simulink model "PC_Quadcopter_Simulation"  (R2020b)
settings: Solver=ode45  StartTime=0.0  StopTime=10  FixedStep=0.05  MaxStep=0.06  RelTol=1e-3  EnableMultiTasking=on
model workspace (MAT data in the model file):
  Sig : Simulink.Signal (value not decoded)
undefined symbols (not defined in the file): IC, quadModel
libraries: pid_lib x9, simulink x6, shared6dof x1
(part 2 of 2)

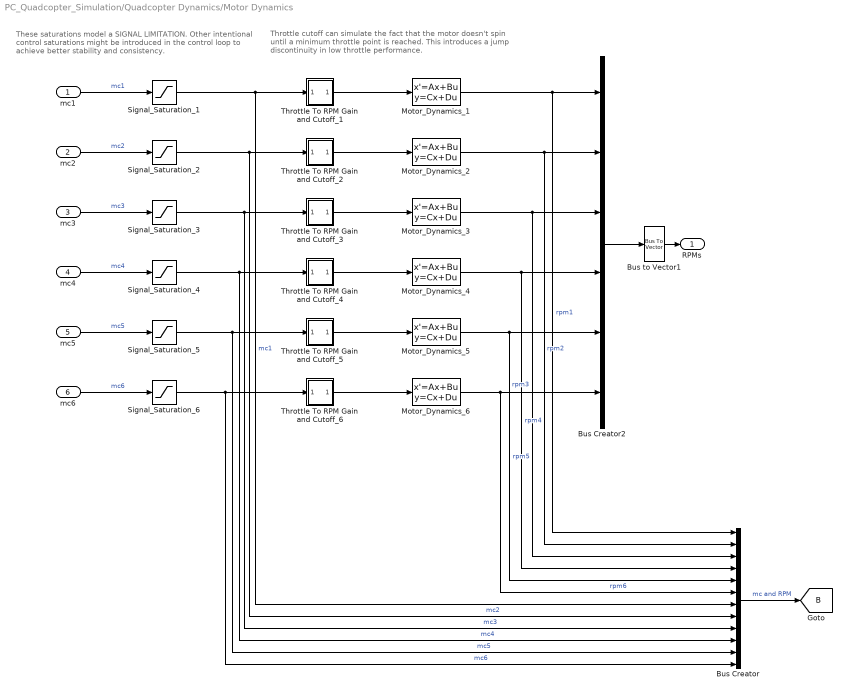
== system PC_Quadcopter_Simulation/Quadcopter Dynamics/Motor Dynamics ==
  note: Throttle cutoff can simulate the fact that the motor doesn't
      | spin until a minimum throttle point is reached. This introduces
      | a jump discontinuity in low throttle performance.
  note: These saturations model a SIGNAL LIMITATION.
      | Other intentional control saturations might be introduced in the
      | control loop to achieve better stability and consistency.
  mc1 : Inport
  mc2 : Inport  Port=2
  mc3 : Inport  Port=3
  mc4 : Inport  Port=4
  mc5 : Inport  Port=5
  mc6 : Inport  Port=6
  Bus Creator : BusCreator  Inputs=12
  Bus Creator2 : BusCreator  Inputs=6
  Bus to Vector1 : BusToVector
  Motor_Dynamics_1 : StateSpace  A=-1/quadModel.T  C=1/quadModel.T  D=0  InitialCondition=IC.w1*quadModel.T
  Motor_Dynamics_2 : StateSpace  A=-1/quadModel.T  C=1/quadModel.T  D=0  InitialCondition=IC.w2*quadModel.T
  Motor_Dynamics_3 : StateSpace  A=-1/quadModel.T  C=1/quadModel.T  D=0  InitialCondition=IC.w3*quadModel.T
  Motor_Dynamics_4 : StateSpace  A=-1/quadModel.T  C=1/quadModel.T  D=0  InitialCondition=IC.w4*quadModel.T
  Motor_Dynamics_5 : StateSpace  A=-1/quadModel.T  C=1/quadModel.T  D=0  InitialCondition=IC.w4*quadModel.T
  Motor_Dynamics_6 : StateSpace  A=-1/quadModel.T  C=1/quadModel.T  D=0  InitialCondition=IC.w4*quadModel.T
  Signal_Saturation_{1..6} (6 alike) : Saturate  UpperLimit=100  LowerLimit=0
  Throttle To RPM Gain and Cutoff_1 : Subsystem
  Throttle To RPM Gain and Cutoff_2 : Subsystem
  Throttle To RPM Gain and Cutoff_3 : Subsystem
  Throttle To RPM Gain and Cutoff_4 : Subsystem
  Throttle To RPM Gain and Cutoff_5 : Subsystem
  Throttle To RPM Gain and Cutoff_6 : Subsystem
  RPMs : Outport
  tag scope: B=global
  wires:
  mc1/1 -> Signal_Saturation_1/1  "mc1"
  mc2/1 -> Signal_Saturation_2/1  "mc2"
  mc3/1 -> Signal_Saturation_3/1  "mc3"
  mc4/1 -> Signal_Saturation_4/1  "mc4"
  Throttle To RPM Gain and Cutoff_1/1(Out5) -> Motor_Dynamics_1/1
  Throttle To RPM Gain and Cutoff_2/1(Out5) -> Motor_Dynamics_2/1
  Throttle To RPM Gain and Cutoff_3/1(Out5) -> Motor_Dynamics_3/1
  Throttle To RPM Gain and Cutoff_4/1(Out5) -> Motor_Dynamics_4/1
  Motor_Dynamics_1/1 -> Bus Creator/1, Bus Creator2/1  "rpm1"
  Motor_Dynamics_2/1 -> Bus Creator/2, Bus Creator2/2  "rpm2"
  Motor_Dynamics_3/1 -> Bus Creator/3, Bus Creator2/3  "rpm3"
  Motor_Dynamics_4/1 -> Bus Creator/4, Bus Creator2/4  "rpm4"
  Bus Creator/1 -> [B]  "mc and RPM"
  mc5/1 -> Signal_Saturation_5/1  "mc5"
  Throttle To RPM Gain and Cutoff_5/1(Out5) -> Motor_Dynamics_5/1
  mc6/1 -> Signal_Saturation_6/1  "mc6"
  Throttle To RPM Gain and Cutoff_6/1(Out5) -> Motor_Dynamics_6/1
  Motor_Dynamics_6/1 -> Bus Creator/6, Bus Creator2/6  "rpm6"
  Motor_Dynamics_5/1 -> Bus Creator/5, Bus Creator2/5  "rpm5"
  Signal_Saturation_3/1 -> Bus Creator/9, Throttle To RPM Gain and Cutoff_3/1(In5)  "mc3"
  Signal_Saturation_4/1 -> Bus Creator/10, Throttle To RPM Gain and Cutoff_4/1(In5)  "mc4"
  Signal_Saturation_1/1 -> Bus Creator/7, Throttle To RPM Gain and Cutoff_1/1(In5)  "mc1"
  Signal_Saturation_5/1 -> Bus Creator/11, Throttle To RPM Gain and Cutoff_5/1(In5)  "mc5"
  Signal_Saturation_6/1 -> Bus Creator/12, Throttle To RPM Gain and Cutoff_6/1(In5)  "mc6"
  Signal_Saturation_2/1 -> Bus Creator/8, Throttle To RPM Gain and Cutoff_2/1(In5)  "mc2"
  Bus Creator2/1 -> Bus to Vector1/1
  Bus to Vector1/1 -> RPMs/1

== system PC_Quadcopter_Simulation/Quadcopter Dynamics/Subsystem ==
  RPMs : Inport
  States : Inport  Port=2
  DCM : Inport  Port=3
  Forces : Subsystem
  Moments : Subsystem
  ForceOut : Outport
  MomentOut : Outport  Port=2
  wires:
  RPMs/1 -> Moments/2(RPMs), Forces/1(RPMs)  "RPMs"
  Forces/1(Forces) -> ForceOut/1
  States/1 -> Moments/1(States)  "States"
  Moments/1(Moments) -> MomentOut/1
  DCM/1 -> Forces/2(DCM)

== system PC_Quadcopter_Simulation/Quadcopter Dynamics/Motor Dynamics/Throttle To RPM Gain and Cutoff_1 ==
  note: minThr should be a quad.mat value
  note: This gain should be a quad.mat value
  note: This constant should be a quad.mat value
  note: Output equals linearly scaled RPM
      | for given throttle input if throttle input >=Throttle Cuttoff (minThr)
      | else output is zero.
  In5 : Inport
  Constant : Constant  Value=quadModel.b
  Gain : Gain  Gain=quadModel.cr
  Minimum Throttle Cutoff : simulink/Logic and Bit Operations/Compare To Constant  relop=>=  const=quadModel.minThr  OutDataTypeStr=uint8
  Product : Product
  Sum1 : Sum  Inputs=++|
  Out5 : Outport
  wires:
  Minimum Throttle Cutoff/1 -> Product/2
  Product/1 -> Out5/1
  In5/1 -> Gain/1, Minimum Throttle Cutoff/1
  Gain/1 -> Sum1/2
  Sum1/1 -> Product/1
  Constant/1 -> Sum1/1

== system PC_Quadcopter_Simulation/Quadcopter Dynamics/Motor Dynamics/Throttle To RPM Gain and Cutoff_2 ==
  note: minThr should be a quad.mat value
  note: This gain should be a quad.mat value
  note: This constant should be a quad.mat value
  note: Output equals linearly scaled RPM
      | for given throttle input if throttle input >=Throttle Cuttoff (minThr)
      | else output is zero.
  In5 : Inport
  Constant : Constant  Value=quadModel.b
  Gain : Gain  Gain=quadModel.cr
  Minimum Throttle Cutoff : simulink/Logic and Bit Operations/Compare To Constant  relop=>=  const=quadModel.minThr  OutDataTypeStr=uint8
  Product : Product
  Sum1 : Sum  Inputs=++|
  Out5 : Outport
  wires:
  Minimum Throttle Cutoff/1 -> Product/2
  Product/1 -> Out5/1
  In5/1 -> Gain/1, Minimum Throttle Cutoff/1
  Gain/1 -> Sum1/2
  Sum1/1 -> Product/1
  Constant/1 -> Sum1/1

== system PC_Quadcopter_Simulation/Quadcopter Dynamics/Motor Dynamics/Throttle To RPM Gain and Cutoff_3 ==
  note: minThr should be a quad.mat value
  note: This gain should be a quad.mat value
  note: This constant should be a quad.mat value
  note: Output equals linearly scaled RPM
      | for given throttle input if throttle input >=Throttle Cuttoff (minThr)
      | else output is zero.
  In5 : Inport
  Constant : Constant  Value=quadModel.b
  Gain : Gain  Gain=quadModel.cr
  Minimum Throttle Cutoff : simulink/Logic and Bit Operations/Compare To Constant  relop=>=  const=quadModel.minThr  OutDataTypeStr=uint8
  Product : Product
  Sum1 : Sum  Inputs=++|
  Out5 : Outport
  wires:
  Minimum Throttle Cutoff/1 -> Product/2
  Product/1 -> Out5/1
  In5/1 -> Gain/1, Minimum Throttle Cutoff/1
  Gain/1 -> Sum1/2
  Sum1/1 -> Product/1
  Constant/1 -> Sum1/1

== system PC_Quadcopter_Simulation/Quadcopter Dynamics/Motor Dynamics/Throttle To RPM Gain and Cutoff_4 ==
  note: minThr should be a quad.mat value
  note: This gain should be a quad.mat value
  note: This constant should be a quad.mat value
  note: Output equals linearly scaled RPM
      | for given throttle input if throttle input >=Throttle Cuttoff (minThr)
      | else output is zero.
  In5 : Inport
  Constant : Constant  Value=quadModel.b
  Gain : Gain  Gain=quadModel.cr
  Minimum Throttle Cutoff : simulink/Logic and Bit Operations/Compare To Constant  relop=>=  const=quadModel.minThr  OutDataTypeStr=uint8
  Product : Product
  Sum1 : Sum  Inputs=++|
  Out5 : Outport
  wires:
  Minimum Throttle Cutoff/1 -> Product/2
  Product/1 -> Out5/1
  In5/1 -> Gain/1, Minimum Throttle Cutoff/1
  Gain/1 -> Sum1/2
  Sum1/1 -> Product/1
  Constant/1 -> Sum1/1

== system PC_Quadcopter_Simulation/Quadcopter Dynamics/Motor Dynamics/Throttle To RPM Gain and Cutoff_5 ==
  note: minThr should be a quad.mat value
  note: This gain should be a quad.mat value
  note: This constant should be a quad.mat value
  note: Output equals linearly scaled RPM
      | for given throttle input if throttle input >=Throttle Cuttoff (minThr)
      | else output is zero.
  In5 : Inport
  Constant : Constant  Value=quadModel.b
  Gain : Gain  Gain=quadModel.cr
  Minimum Throttle Cutoff : simulink/Logic and Bit Operations/Compare To Constant  relop=>=  const=quadModel.minThr  OutDataTypeStr=uint8
  Product : Product
  Sum1 : Sum  Inputs=++|
  Out5 : Outport
  wires:
  Minimum Throttle Cutoff/1 -> Product/2
  Product/1 -> Out5/1
  In5/1 -> Gain/1, Minimum Throttle Cutoff/1
  Gain/1 -> Sum1/2
  Sum1/1 -> Product/1
  Constant/1 -> Sum1/1

== system PC_Quadcopter_Simulation/Quadcopter Dynamics/Motor Dynamics/Throttle To RPM Gain and Cutoff_6 ==
  note: minThr should be a quad.mat value
  note: This gain should be a quad.mat value
  note: This constant should be a quad.mat value
  note: Output equals linearly scaled RPM
      | for given throttle input if throttle input >=Throttle Cuttoff (minThr)
      | else output is zero.
  In5 : Inport
  Constant : Constant  Value=quadModel.b
  Gain : Gain  Gain=quadModel.cr
  Minimum Throttle Cutoff : simulink/Logic and Bit Operations/Compare To Constant  relop=>=  const=quadModel.minThr  OutDataTypeStr=uint8
  Product : Product
  Sum1 : Sum  Inputs=++|
  Out5 : Outport
  wires:
  Minimum Throttle Cutoff/1 -> Product/2
  Product/1 -> Out5/1
  In5/1 -> Gain/1, Minimum Throttle Cutoff/1
  Gain/1 -> Sum1/2
  Sum1/1 -> Product/1
  Constant/1 -> Sum1/1

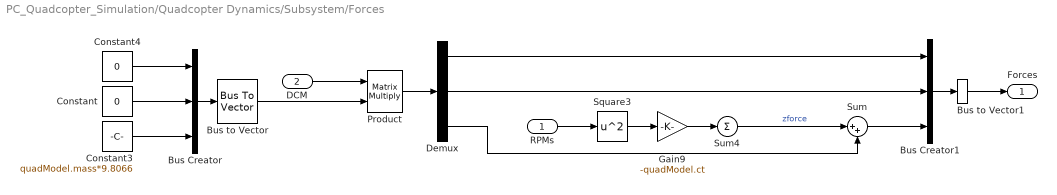
== system PC_Quadcopter_Simulation/Quadcopter Dynamics/Subsystem/Forces ==
  RPMs : Inport
  DCM : Inport  Port=2
  Bus Creator : BusCreator  Inputs=3
  Bus Creator1 : BusCreator  Inputs=3
  Bus to Vector : BusToVector
  Bus to Vector1 : BusToVector
  Constant : Constant  Value=0
  Constant3 : Constant  Value=quadModel.mass*9.8066
  Constant4 : Constant  Value=0
  Demux : Demux  Outputs=3
  Gain9 : Gain  Gain=-quadModel.ct
  Product : Product  Multiplication=Matrix(*)
  Square3 : Math  Operator=square  SaturateOnIntegerOverflow=on
  Sum : Sum  Inputs=|++
  Sum4 : Sum  Inputs=+
  Forces : Outport
  wires:
  Demux/2 -> Bus Creator1/2
  Bus Creator1/1 -> Bus to Vector1/1
  Demux/1 -> Bus Creator1/1
  Gain9/1 -> Sum4/1
  Bus to Vector1/1 -> Forces/1
  Square3/1 -> Gain9/1
  Sum4/1 -> Sum/1  "zforce"
  RPMs/1 -> Square3/1
  DCM/1 -> Product/1
  Constant4/1 -> Bus Creator/1
  Constant/1 -> Bus Creator/2
  Bus Creator/1 -> Bus to Vector/1
  Constant3/1 -> Bus Creator/3
  Bus to Vector/1 -> Product/2
  Product/1 -> Demux/1
  Sum/1 -> Bus Creator1/3
  Demux/3 -> Sum/2

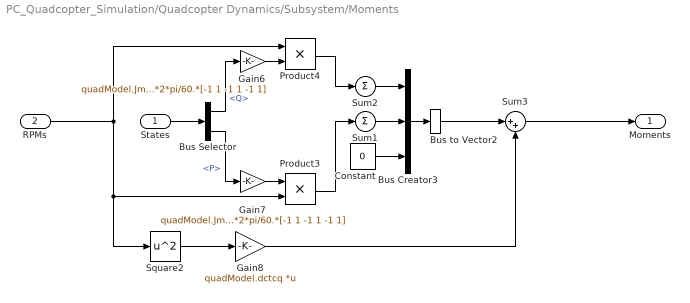
== system PC_Quadcopter_Simulation/Quadcopter Dynamics/Subsystem/Moments ==
  States : Inport
  RPMs : Inport  Port=2
  Bus Creator3 : BusCreator  Inputs=3
  Bus Selector : BusSelector  OutputSignals=Q,P
  Bus to Vector2 : BusToVector
  Constant : Constant  Value=0
  Gain6 : Gain  Gain=quadModel.Jm*2*pi/60.*[-1 1 -1 1 -1 1]
  Gain7 : Gain  Gain=quadModel.Jm*2*pi/60.*[-1 1 -1 1 -1 1]
  Gain8 : Gain  Gain=quadModel.dctcq  Multiplication=Matrix(K*u)
  Product3 : Product
  Product4 : Product
  Square2 : Math  Operator=square  SaturateOnIntegerOverflow=on
  Sum1 : Sum  Inputs=+
  Sum2 : Sum  Inputs=+
  Sum3 : Sum  Inputs=|++
  Moments : Outport
  wires:
  Sum1/1 -> Bus Creator3/2
  Bus Selector/1 -> Gain6/1  "<Q>"
  Bus to Vector2/1 -> Sum3/1
  Product4/1 -> Sum2/1
  Constant/1 -> Bus Creator3/3
  Gain6/1 -> Product4/2
  Bus Selector/2 -> Gain7/1  "<P>"
  Gain7/1 -> Product3/1
  RPMs/1 -> Product4/1, Product3/2, Square2/1
  Sum2/1 -> Bus Creator3/1
  Bus Creator3/1 -> Bus to Vector2/1
  Gain8/1 -> Sum3/2
  Product3/1 -> Sum1/1
  Square2/1 -> Gain8/1
  Sum3/1 -> Moments/1
  States/1 -> Bus Selector/1
